simulink library "INT_VehV_DD"  (R2016b)
settings: Solver=VariableStepAuto  StartTime=0.0  StopTime=10.0  RelTol=1e-3
settings Model: Creator=Administrator  LastModifiedBy=Administrator

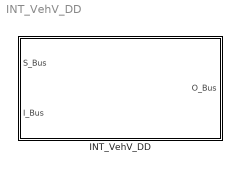
== system INT_VehV_DD ==
  INT_VehV_DD : Subsystem

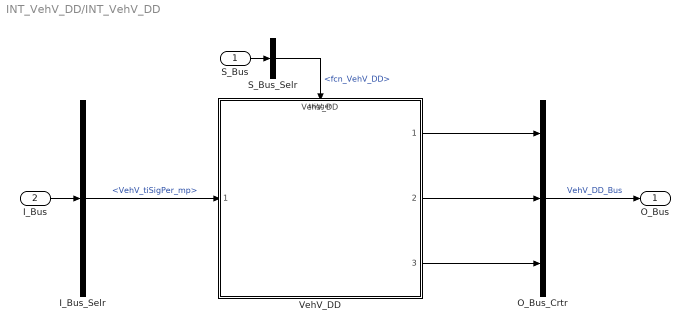
== system INT_VehV_DD/INT_VehV_DD ==
  S_Bus : Inport
  I_Bus : Inport  Port=2
  I_Bus_Selr : BusSelector  OutputSignals=VehV_tiSigPer_mp
  O_Bus_Crtr : BusCreator  Inputs=3
  S_Bus_Selr : BusSelector  OutputSignals=fcn_VehV_DD
  VehV_DD : ModelReference  ModelNameDialog=VehV_DD  SimulationMode=Normal  ModelReferenceVersion=1.5  TriggerPortName=function  TriggerPortTriggerType=function-call  TriggerPortStatesWhenEnabling=held
  O_Bus : Outport
  wires:
  S_Bus_Selr/1 -> VehV_DD/Trigger  "<fcn_VehV_DD>"
  S_Bus/1 -> S_Bus_Selr/1
  I_Bus/1 -> I_Bus_Selr/1
  I_Bus_Selr/1 -> VehV_DD/1  "<VehV_tiSigPer_mp>"
  O_Bus_Crtr/1 -> O_Bus/1  "VehV_DD_Bus"
  VehV_DD/1 -> O_Bus_Crtr/1
  VehV_DD/2 -> O_Bus_Crtr/2
  VehV_DD/3 -> O_Bus_Crtr/3
